simulink model "bldc"  (R2020a)
settings: Solver=VariableStepAuto  StartTime=0.0  StopTime=3  RelTol=1e-3
settings Model: Creator=Admin  LastModifiedBy=Admin

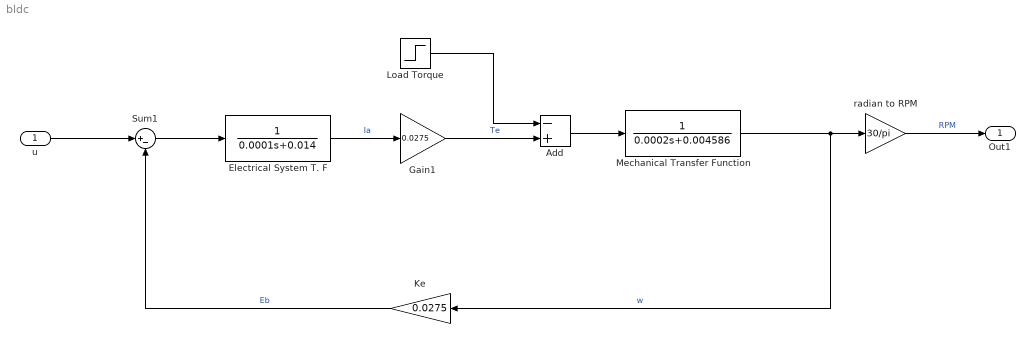
== system bldc ==
  u : Inport
  Add : Sum  Inputs=-+
  Electrical System T. F : TransferFcn  Denominator=[0.0001 0.014]
  Gain1 : Gain  Gain=0.0275
  Ke : Gain  Gain=0.0275
  Load Torque : Step  After=10  SampleTime=0
  Mechanical Transfer Function : TransferFcn  Denominator=[0.0002 0.004586]
  Sum1 : Sum  Inputs=|+-
  radian to RPM : Gain  Gain=30/pi
  Out1 : Outport
  wires:
  Mechanical Transfer Function/1 -> Ke/1, radian to RPM/1  "w"
  Gain1/1 -> Add/2  "Te"
  Ke/1 -> Sum1/2  "Eb"
  Sum1/1 -> Electrical System T. F/1
  radian to RPM/1 -> Out1/1  "RPM"
  u/1 -> Sum1/1
  Load Torque/1 -> Add/1
  Add/1 -> Mechanical Transfer Function/1
  Electrical System T. F/1 -> Gain1/1  "Ia"
